simulink model "intento1"  (R2017b)
settings: Solver=VariableStepAuto  StartTime=0.0  StopTime=1  RelTol=1e-3
values from neighbouring files (symbols this model uses):
  kd = eval(S.kd)    [Lab4.m]    (also in Lab4Final.m; Lab4intento2.m; Lab4intento3.m)
  kd2 = eval(S.kd2)    [Lab4.m]    (also in Lab4Final.m; Lab4intento3.m)
  kd3 = eval(S.kd3)    [Lab4.m]    (also in Lab4intento3.m)
  ki = eval(S.ki)    [Lab4.m]    (also in Lab4Final.m; Lab4intento2.m; Lab4intento3.m)
  kp = eval(S.kp)    [Lab4.m]    (also in Lab4Final.m; Lab4intento2.m; Lab4intento3.m)
settings Model: Creator=Cx001la  LastModifiedBy=Cx001la

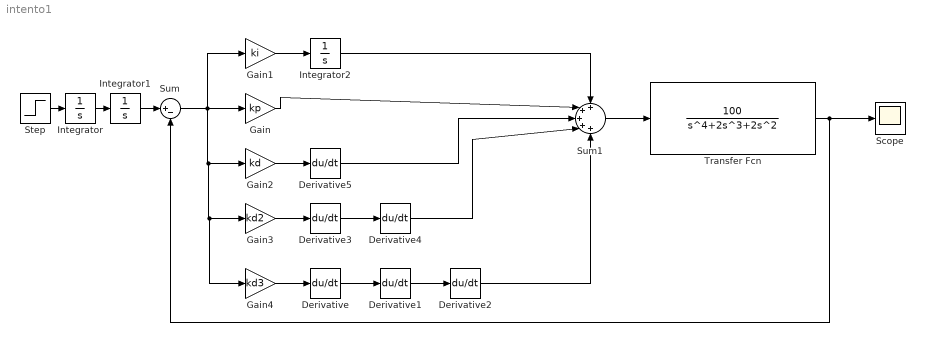
== system intento1 ==
  Derivative{,1..5} (6 alike) : Derivative
  Gain : Gain  Gain=kp
  Gain1 : Gain  Gain=ki
  Gain2 : Gain  Gain=kd
  Gain3 : Gain  Gain=kd2
  Gain4 : Gain  Gain=kd3
  Integrator : Integrator
  Integrator1 : Integrator
  Integrator2 : Integrator
  Scope : Scope
  Step : Step  Time=0  SampleTime=0
  Sum : Sum  Inputs=|+-
  Sum1 : Sum  Inputs=+++++
  Transfer Fcn : TransferFcn  Numerator=[100]  Denominator=[1 2 2 0 0]
  wires:
  Step/1 -> Integrator/1
  Integrator/1 -> Integrator1/1
  Integrator1/1 -> Sum/1
  Sum/1 -> Gain1/1, Gain4/1, Gain3/1, Gain2/1, Gain/1
  Gain4/1 -> Derivative/1
  Derivative/1 -> Derivative1/1
  Derivative1/1 -> Derivative2/1
  Derivative3/1 -> Derivative4/1
  Gain3/1 -> Derivative3/1
  Gain2/1 -> Derivative5/1
  Gain1/1 -> Integrator2/1
  Integrator2/1 -> Sum1/1
  Gain/1 -> Sum1/2
  Derivative5/1 -> Sum1/3
  Derivative4/1 -> Sum1/4
  Derivative2/1 -> Sum1/5
  Sum1/1 -> Transfer Fcn/1
  Transfer Fcn/1 -> Scope/1, Sum/2
